simulink model "project_2_sim"  (R2025b)
settings: Solver=VariableStepAuto  StartTime=0.0  StopTime=10.0  RelTol=1e-3
settings Model: Creator=chris  LastModifiedBy=chris

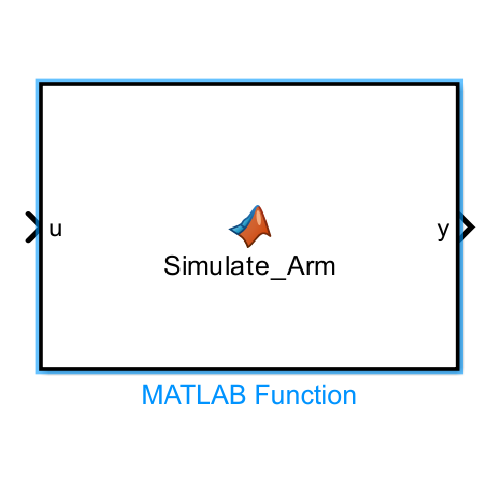
[thumbnail: Simulink's stored preview of the top-level diagram]
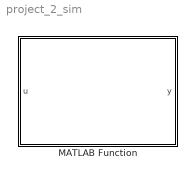
== system project_2_sim ==
  MATLAB Function : MATLAB Function  Description=Simulate_SF  TreatAsAtomicUnit=on

== matlab function project_2_sim/MATLAB Function ==
  data: u input; y output
function y = Simulate_Arm(u)

y = u;
